simulink model "model_verification"  (Simulink 6.3)
settings: Solver=ode45  StartTime=0.0  StopTime=6174  RelTol=1e-3
InitFcn:
  | model_veri
undefined symbols (not defined in the file): A_model_ver, B_model_ver, C_model_ver, D_model_ver, maxTorque
libraries: components_lib x10, simulink x5
settings Model: Creator=krage  LastModifiedBy=mnkr02  ExtModeAutoUpdateStatusClock=off  StrictBusMsg=None
settings DebuggingCC: CheckSSInitialOutputMsg=off

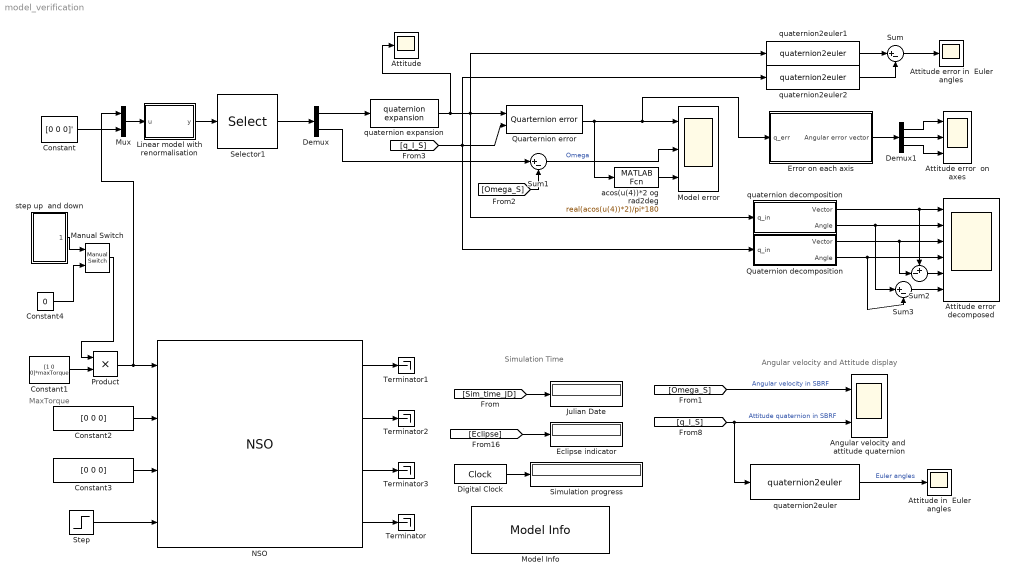
== system model_verification ==
  note: Simulation Time
  note: Angular velocity and Attitude display
  note: MaxTorque
  Angular velocity and  attitude quaternion : Scope  NumInputPorts=2
      settings: YMin=-1.25e-008~0  YMax=0~1
  Attitude : Scope
      settings: YMin=-3.5  YMax=3.5  SaveName=ScopeData2
  Attitude error  decomposed : Scope  NumInputPorts=6
      settings: YMin=-1~0~-1~0~-0.001~-5e-010  YMax=0.1~0.00125~1~0.00125~0.01~2.5e-009  SaveName=ScopeData4
  Attitude error  on axes : Scope  NumInputPorts=3
      settings: YMin=-3.5~-5~-5  YMax=3.5~5~5  SaveName=ScopeData5
  Attitude error in  Euler angles : Scope
      settings: YMin=-3.5  YMax=3.5  SaveName=ScopeData3
  Attitude in  Euler angles : Scope
      settings: YMin=-3.5  YMax=3.5
  Constant : Constant  Value=[0 0 0]'
  Constant1 : Constant  Value=[1 0 0]*maxTorque
  Constant2 : Constant  Value=[0 0 0]
  Constant3 : Constant  Value=[0 0 0]
  Constant4 : Constant  Value=0
  Demux : Demux  Outputs=2
  Demux1 : Demux  Outputs=3
  Digital Clock : DigitalClock
  Eclipse indicator : Display
  Error on each axis : Subsystem
  Julian Date : Display
  Linear model with renormalisation : Subsystem  mask(Linear satellite system){Asat=A_model_ver, Bsat=B_model_ver, Csat=C_model_ver, Dsat=D_model_ver, q_init=[0 0 0 1], w_init=[0.1 0.1 0.1]*0}
      mask prompts: Asat "A matrix"; Bsat "B matrix"; Csat "C matrix"; Dsat "D matrix"; q_init "Initial attitude"; w_init "Initial angular rate"
      mask help:
      | This is a general linear system of a satellite described by
      | x_dot = Ax + Bu
      | y = Cx + Du
      | where x = [q_1:3 w L] and u=[N_mt N_mw].
      | However, in this model the quaternion is expanded and renormalised in every timestep.
  Manual Switch : simulink/Signal Routing/Manual Switch  sw=1  action=0
  Model Info : simulink/Model-Wide Utilities/Model Info  InitialBlockCM=None  BlockCM=None  Frame=on  DisplayStringWithTags=|  HorizontalTextAlignment=Left  LeftAlignmentValue=0.02  SourceBlockDiagram=model_verification  TagMaxNumber=20
      | Usefull Julian dates:
      | sun to eclipse : 2452315.560376
      | 32 sec. before : 2452315.56
      | eclipse to sun : 2452315.513363
  Model error : Scope  NumInputPorts=3
      settings: TimeRange=8.824896694214885  YMin=-1~-1e-016~0  YMax=1~2e-016~0.4935266347021195  SaveName=model_veri_err
  Mux : Mux  Inputs=2
  NSO : components_lib/NSO  Tag=AAUSAT-II Model  Description=AAUSAT-II Model  r_com_s=[0.05 0.05 0.15]  sat_temp_start=0  r_com_s_deployed=[0.05 0.05 0.125]  mass_sc=3  Dim=[0.1 0.1 0.3]  inertia_c=[25 25 5]/1e3  inertia_d=[42.3 42.3 28.4]/1e3  init_jd=2452315.56  q_s_c=[0 0 0 1]  q_init_s_i=[0 0 0 1]  w_init_s=[0.1 0.1 0.1]*0  Cd=2  rho=9.25e-13  enable_sensor_emulation=off  alb_emu_enabled=off  enable_dist=off
  Product : Product  RndMeth=Zero
  Quarternion error : components_lib/Math utilities/Quaternion operations/Quarternion error
  Quaternion decomposition : Subsystem
  Selector1 : Selector  Elements=[1 2 3 4 5 6]  InputPortWidth=9
  Simulation progress : Display
  Step : Step  Time=0  SampleTime=0
  Sum : Sum  Inputs=|+-
  Sum1 : Sum  Inputs=|+-
  Sum2 : Sum  Inputs=+-|
  Sum3 : Sum  Inputs=|+-
  Terminator{,1..3} (4 alike) : Terminator
  acos(u(4))*2 og rad2deg : MATLABFcn  MATLABFcn=real(acos(u(4))*2)/pi*180
  quaternion decomposition : Subsystem
  quaternion expansion : components_lib/Math utilities/Quaternion operations/quaternion expansion
  quaternion2euler : components_lib/Math utilities/Quaternion operations/quaternion2euler
  quaternion2euler1 : components_lib/Math utilities/Quaternion operations/quaternion2euler
  quaternion2euler2 : components_lib/Math utilities/Quaternion operations/quaternion2euler
  step up  and down : Subsystem  mask{up_start_time=300, up_end_time=320, down_start_time=1300, down_end_time=1320}
      mask prompts: up_start_time "Pulse up start time"; up_end_time "Pulse up end time"; down_start_time "Pulse down start time"; down_end_time "Pulse down end time"
      mask help: Gives first a positive pulse of size 1 and then a negative pulse of size 1.
  wires:
  [Omega_S] -> Angular velocity and  attitude quaternion/1  "Angular velocity in SBRF"
  [q_I_S] -> quaternion2euler/1, Angular velocity and  attitude quaternion/2  "Attitude quaternion in SBRF"
  quaternion2euler/1 -> Attitude in  Euler angles/1  "Euler angles"
  [Sim_time_JD] -> Julian Date/1
  [Eclipse] -> Eclipse indicator/1
  Digital Clock/1 -> Simulation progress/1
  Step/1 -> NSO/4
  NSO/1 -> Terminator1/1
  NSO/2 -> Terminator2/1
  NSO/3 -> Terminator3/1
  NSO/4 -> Terminator/1
  Constant2/1 -> NSO/2
  Constant3/1 -> NSO/3
  Sum1/1 -> Model error/2  "Omega"
  Constant/1 -> Mux/2
  [Omega_S] -> Sum1/2
  Demux/2 -> Sum1/1
  Selector1/1 -> Demux/1
  Quarternion error/1 -> acos(u(4))*2 og rad2deg/1, Model error/1, Error on each axis/1(q_err)
  quaternion expansion/1 -> Quarternion error/1, quaternion2euler1/1, quaternion decomposition/1(q_in), Attitude/1
  [q_I_S] -> Quarternion error/2, quaternion2euler2/1, Quaternion decomposition/1(q_in)
  quaternion2euler2/1 -> Sum/2
  quaternion2euler1/1 -> Sum/1
  Sum/1 -> Attitude error in  Euler angles/1
  quaternion decomposition/1(Vector) -> Attitude error  decomposed/1, Sum2/1
  quaternion decomposition/2(Angle) -> Attitude error  decomposed/2, Sum3/1
  Quaternion decomposition/1(Vector) -> Attitude error  decomposed/3, Sum2/2
  Quaternion decomposition/2(Angle) -> Attitude error  decomposed/4, Sum3/2
  Sum2/1 -> Attitude error  decomposed/5
  Sum3/1 -> Attitude error  decomposed/6
  acos(u(4))*2 og rad2deg/1 -> Model error/3
  Product/1 -> NSO/1, Mux/1
  Constant1/1 -> Product/2
  Constant4/1 -> Manual Switch/2
  Manual Switch/1 -> Product/1
  Error on each axis/1(Angular error vector) -> Demux1/1
  Demux1/1 -> Attitude error  on axes/1
  Demux1/2 -> Attitude error  on axes/2
  Demux1/3 -> Attitude error  on axes/3
  Mux/1 -> Linear model with renormalisation/1(u)
  Linear model with renormalisation/1(y) -> Selector1/1
  step up  and down/1(Signal) -> Manual Switch/1
  Demux/1 -> quaternion expansion/1

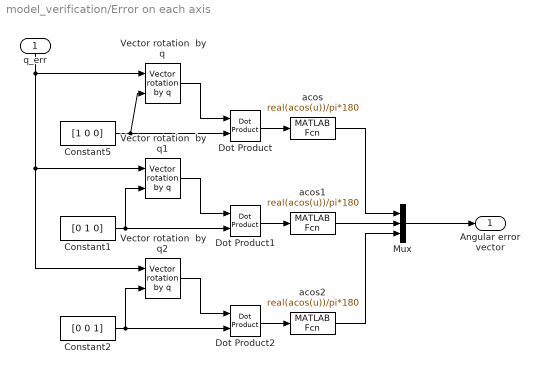
== system model_verification/Error on each axis ==
  q_err : Inport  Orientation=down
  Constant1 : Constant  Value=[0 1 0]
  Constant2 : Constant  Value=[0 0 1]
  Constant5 : Constant  Value=[1 0 0]
  Dot Product : simulink/Math Operations/Dot Product  InputSameDT=on  OutDataType=sfix(16)  OutScaling=2^-10  DoSatur=off
  Dot Product1 : simulink/Math Operations/Dot Product  InputSameDT=on  OutDataType=sfix(16)  OutScaling=2^-10  DoSatur=off
  Dot Product2 : simulink/Math Operations/Dot Product  InputSameDT=on  OutDataType=sfix(16)  OutScaling=2^-10  DoSatur=off
  Mux : Mux  Inputs=3
  Vector rotation  by q : components_lib/Math utilities/Quaternion operations/Vector rotation by q
  Vector rotation  by q1 : components_lib/Math utilities/Quaternion operations/Vector rotation by q
  Vector rotation  by q2 : components_lib/Math utilities/Quaternion operations/Vector rotation by q
  acos : MATLABFcn  MATLABFcn=real(acos(u))/pi*180
  acos1 : MATLABFcn  MATLABFcn=real(acos(u))/pi*180
  acos2 : MATLABFcn  MATLABFcn=real(acos(u))/pi*180
  Angular error vector : Outport
  wires:
  Constant5/1 -> Dot Product/2, Vector rotation  by q/2
  Vector rotation  by q/1 -> Dot Product/1
  Dot Product/1 -> acos/1
  q_err/1 -> Vector rotation  by q/1, Vector rotation  by q1/1, Vector rotation  by q2/1
  Constant1/1 -> Vector rotation  by q1/2, Dot Product1/2
  Vector rotation  by q1/1 -> Dot Product1/1
  Dot Product1/1 -> acos1/1
  Constant2/1 -> Vector rotation  by q2/2, Dot Product2/2
  Vector rotation  by q2/1 -> Dot Product2/1
  Dot Product2/1 -> acos2/1
  acos/1 -> Mux/1
  acos1/1 -> Mux/2
  acos2/1 -> Mux/3
  Mux/1 -> Angular error vector/1

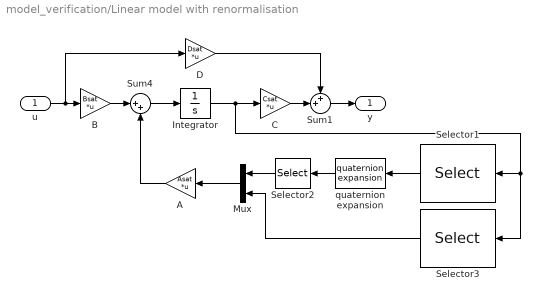
== system model_verification/Linear model with renormalisation ==
  u : Inport
  A : Gain  Orientation=left  Gain=Asat  Multiplication=Matrix(K*u)
  B : Gain  Gain=Bsat  Multiplication=Matrix(K*u)
  C : Gain  Gain=Csat  Multiplication=Matrix(K*u)
  D : Gain  Gain=Dsat  Multiplication=Matrix(K*u)
  Integrator : Integrator  InitialCondition=[q_init(1:3) w_init 0 0 0]
  Mux : Mux  Orientation=left  Inputs=2
  Selector1 : Selector  Orientation=left  Elements=[1 2 3]  InputPortWidth=9
  Selector2 : Selector  Orientation=left  Elements=[1 2 3]  InputPortWidth=4
  Selector3 : Selector  Orientation=left  Elements=[4 5 6 7 8 9]  InputPortWidth=9
  Sum1 : Sum  Inputs=++|
  Sum4 : Sum  Inputs=|++
  quaternion expansion : components_lib/Math utilities/Quaternion operations/quaternion expansion  Orientation=left
  y : Outport
  wires:
  B/1 -> Sum4/1
  Sum4/1 -> Integrator/1
  Integrator/1 -> C/1, Selector1/1, Selector3/1
  u/1 -> B/1, D/1
  A/1 -> Sum4/2
  D/1 -> Sum1/1
  C/1 -> Sum1/2
  Sum1/1 -> y/1
  Selector1/1 -> quaternion expansion/1
  quaternion expansion/1 -> Selector2/1
  Selector2/1 -> Mux/1
  Selector3/1 -> Mux/2
  Mux/1 -> A/1

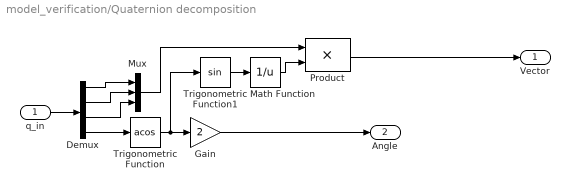
== system model_verification/Quaternion decomposition ==
  q_in : Inport
  Demux : Demux
  Gain : Gain  Gain=2  SaturateOnIntegerOverflow=on
  Math Function : Math  Operator=reciprocal  SaturateOnIntegerOverflow=on
  Mux : Mux  Inputs=3
  Product : Product  SaturateOnIntegerOverflow=on
  Trigonometric Function : Trigonometry  Operator=acos
  Trigonometric Function1 : Trigonometry
  Vector : Outport
  Angle : Outport  Port=2
  wires:
  Product/1 -> Vector/1
  Trigonometric Function1/1 -> Math Function/1
  Math Function/1 -> Product/2
  Mux/1 -> Product/1
  Demux/3 -> Mux/3
  Demux/2 -> Mux/2
  Demux/1 -> Mux/1
  Gain/1 -> Angle/1
  Trigonometric Function/1 -> Trigonometric Function1/1, Gain/1
  Demux/4 -> Trigonometric Function/1
  q_in/1 -> Demux/1

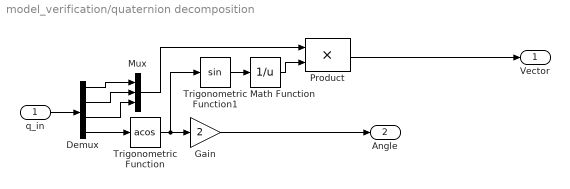
== system model_verification/quaternion decomposition ==
  q_in : Inport
  Demux : Demux
  Gain : Gain  Gain=2  SaturateOnIntegerOverflow=on
  Math Function : Math  Operator=reciprocal  SaturateOnIntegerOverflow=on
  Mux : Mux  Inputs=3
  Product : Product  SaturateOnIntegerOverflow=on
  Trigonometric Function : Trigonometry  Operator=acos
  Trigonometric Function1 : Trigonometry
  Vector : Outport
  Angle : Outport  Port=2
  wires:
  Product/1 -> Vector/1
  Trigonometric Function1/1 -> Math Function/1
  Math Function/1 -> Product/2
  Mux/1 -> Product/1
  Demux/3 -> Mux/3
  Demux/2 -> Mux/2
  Demux/1 -> Mux/1
  Gain/1 -> Angle/1
  Trigonometric Function/1 -> Trigonometric Function1/1, Gain/1
  Demux/4 -> Trigonometric Function/1
  q_in/1 -> Demux/1

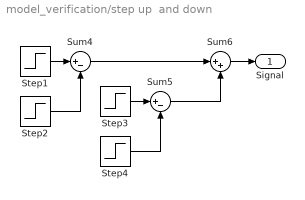
== system model_verification/step up  and down ==
  Step1 : Step  Time=up_start_time  SampleTime=0
  Step2 : Step  Time=up_end_time  SampleTime=0
  Step3 : Step  Time=down_start_time  After=-1  SampleTime=0
  Step4 : Step  Time=down_end_time  After=-1  SampleTime=0
  Sum4 : Sum  Inputs=|+-
  Sum5 : Sum  Inputs=|+-
  Sum6 : Sum  Inputs=|++
  Signal : Outport
  wires:
  Step1/1 -> Sum4/1
  Step2/1 -> Sum4/2
  Step3/1 -> Sum5/1
  Step4/1 -> Sum5/2
  Sum4/1 -> Sum6/1
  Sum5/1 -> Sum6/2
  Sum6/1 -> Signal/1
